simulink library "SuperLogic"  (Simulink 7.0)
libraries: RT x1
settings Model: Creator=ugur  LastModifiedBy=xx

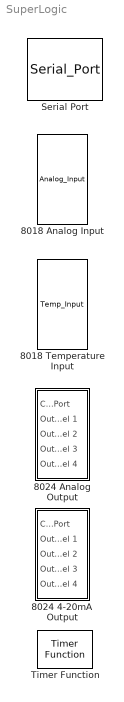
== system SuperLogic ==
  8018 Analog Input : S-Function  FunctionName=Analog_Input  Parameters=AC1, AC2, AC3, AC4, AC5, AC6, AC7, AC8  mask(S function: Analog Input){AC1=on, AC2=off, AC3=off, AC4=off, AC5=off, AC6=off, AC7=off, AC8=off}
      mask prompts: AC1 "Analog Channel 1"; AC2 "Analog Channel 2"; AC3 "Analog Channel 3"; AC4 "Analog Channel 4"; AC5 "Analog Channel 5"; AC6 "Analog Channel 6"; AC7 "Analog Channel 7"; AC8 "Analog Channel 8"
      mask help:
      | This M-file reads the analog input channels from the SL 8018 with 8520
      | The first input is the Com_port number from Serial Port Block.
      mask Display: image(imread('8018.jpg'))
  8018 Temperature Input : S-Function  FunctionName=Temp_Input  Parameters=TC1, TC2, TC3, TC4, TC5, TC6, TC7, TC8  mask(S function: Temperature Input){TC1=on, TC2=off, TC3=off, TC4=off, TC5=off, TC6=off, TC7=off, TC8=off}
      mask prompts: TC1 "Temperature Channel 1"; TC2 "Temperature Channel 2"; TC3 "Temperature Channel 3"; TC4 "Temperature Channel 4"; TC5 "Temperature Channel 5"; TC6 "Temperature Channel 6"; TC7 "Temperature Channel 7"; TC8 "Temperature Channel 8"
      mask help:
      | This M-file reads the temperature input channels from the SL 8018 with 8520
      | The first input is the Com_port number from Serial Port Block.
      mask Display: image(imread('8018.jpg'))
  8024 4-20mA Output : Subsystem  TreatAsAtomicUnit=on  mask(S function: Analog Output){OC1=on, OC2=off, OC3=off, OC4=off}
      mask prompts: OC1 "Output Channel 1"; OC2 "Output Channel 2"; OC3 "Output Channel 3"; OC4 "Output Channel 4"
      mask help:
      | This M-file sets the analog output channels from the SL 8024 with 8520
      | The first input is the Com_port number from Serial Port Block.
      mask Display: image(imread('8018.jpg'))
  8024 Analog Output : Subsystem  TreatAsAtomicUnit=on  mask(S function: Analog Output){OC1=on, OC2=off, OC3=off, OC4=off}
      mask prompts: OC1 "Output Channel 1"; OC2 "Output Channel 2"; OC3 "Output Channel 3"; OC4 "Output Channel 4"
      mask help:
      | This M-file sets the analog output channels from the SL 8024 with 8520
      | The first input is the Com_port number from Serial Port Block.
      mask Display: image(imread('8018.jpg'))
  Serial Port : S-Function  FunctionName=Serial_Port  Parameters=PORT_NAME, PORT_BRATE  mask(S function : Comm Port ){PORT_NAME=COM1, PORT_BRATE=19200}
      mask prompts: PORT_NAME "Port"; PORT_BRATE "BaudRate"
      mask help:
      | Opens and initializes the selected COM port with the
      | selected parameters at the start of the simulation. At the termination
      | of the simulation closes the COM port and destroy the handle.
      |
      | The output of the block is the handle to the Com port.
      mask StyleString: popup(COM1|COM2|COM3|COM4),popup(4800|9600|19200|38400|57600|115200)
      mask Display: image(imread('dsub9.jpg'))
  Timer Function : RT/Timer Function  step=50  tmrpriority=HIGH  ThPriority=TIME CRITICAL

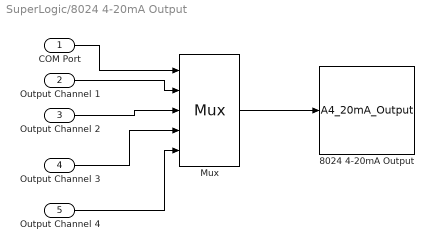
== system SuperLogic/8024 4-20mA Output ==
  COM Port : Inport  OutDataType=sfix(16)  OutScaling=2^0
  Output Channel 1 : Inport  Port=2  OutDataType=sfix(16)  OutScaling=2^0
  Output Channel 2 : Inport  Port=3  OutDataType=sfix(16)  OutScaling=2^0
  Output Channel 3 : Inport  Port=4  OutDataType=sfix(16)  OutScaling=2^0
  Output Channel 4 : Inport  Port=5  OutDataType=sfix(16)  OutScaling=2^0
  8024 4-20mA Output : S-Function  FunctionName=A4_20mA_Output  Parameters=OC1, OC2, OC3, OC4
  Mux : Mux  Inputs=5
      settings: DisplayOption=signals
  wires:
  Output Channel 4/1 -> Mux/5
  Output Channel 3/1 -> Mux/4
  Output Channel 2/1 -> Mux/3
  Output Channel 1/1 -> Mux/2
  COM Port/1 -> Mux/1
  Mux/1 -> 8024 4-20mA Output/1

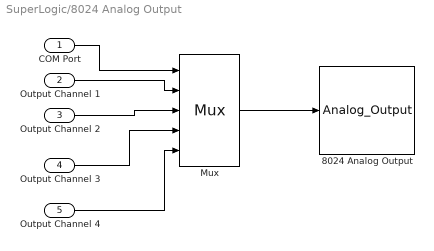
== system SuperLogic/8024 Analog Output ==
  COM Port : Inport  OutDataType=sfix(16)  OutScaling=2^0
  Output Channel 1 : Inport  Port=2  OutDataType=sfix(16)  OutScaling=2^0
  Output Channel 2 : Inport  Port=3  OutDataType=sfix(16)  OutScaling=2^0
  Output Channel 3 : Inport  Port=4  OutDataType=sfix(16)  OutScaling=2^0
  Output Channel 4 : Inport  Port=5  OutDataType=sfix(16)  OutScaling=2^0
  8024 Analog Output : S-Function  FunctionName=Analog_Output  Parameters=OC1, OC2, OC3, OC4
  Mux : Mux  Inputs=5
      settings: DisplayOption=signals
  wires:
  Mux/1 -> 8024 Analog Output/1
  COM Port/1 -> Mux/1
  Output Channel 1/1 -> Mux/2
  Output Channel 2/1 -> Mux/3
  Output Channel 3/1 -> Mux/4
  Output Channel 4/1 -> Mux/5
